simulink model "TV2016"  (Simulink 8.5)
settings: Solver=FixedStepDiscrete  StartTime=0.0  StopTime=inf  FixedStep=0.001  RelTol=1e-3
PreLoadFcn:
  | FSE_Parameters
values from neighbouring files (symbols this model uses):
  car_params = Simulink_Car_params    [TV2016_parameters.m]
  i_Diff = 15.47    [TV2016_parameters.m]
  Kp = 1    [TV2016_parameters.m]
  powerLimitControl = Simulink_el    [TV2016_parameters.m]
  settings = Simulink_Settings    [TV2016_parameters.m]
  SpdC_BCC = 0    [TV2016_parameters.m]
  Speed_Neg_sat = -21    [TV2016_parameters.m]
  Speed_Pos_sat = 21    [TV2016_parameters.m]
  speedEstimation = Simulink_speedEst    [TV2016_parameters.m]
  Tn_n = 0    [TV2016_parameters.m]
  tractionControl = Simulink_tc    [TV2016_parameters.m]
  Use_Joystick = 1    [TV2016_parameters.m]
  yawRateControl = Simulink_yawRate    [TV2016_parameters.m]
libraries: CarMaker4SL x174, simulink x27, simulink_extras x14
(part 4 of 5)

== system TV2016/CarMaker/IPG Vehicle/CarAndTrailer/Trailer/CreateBus Vhcl.Wheel.RR ==
  In1 : Inport
  Bus Creator3 : BusCreator  Inputs=14
  Demux3 : Demux  Outputs=14
  Out1 : Outport
  wires:
  Demux3/14 -> Bus Creator3/14  "Vhcl Wheel RR Trq_WhlBearing"
  Demux3/13 -> Bus Creator3/13  "Vhcl Wheel RR Trq_T2W"
  Demux3/12 -> Bus Creator3/12  "Vhcl Wheel RR SideSlip"
  Demux3/11 -> Bus Creator3/11  "Vhcl Wheel RR LongSlip"
  Demux3/10 -> Bus Creator3/10  "Vhcl Wheel RR vBelt"
  Demux3/9 -> Bus Creator3/9  "Vhcl Wheel RR Fz"
  Demux3/8 -> Bus Creator3/8  "Vhcl Wheel RR Fy"
  Demux3/7 -> Bus Creator3/7  "Vhcl Wheel RR Fx"
  Demux3/6 -> Bus Creator3/6  "Vhcl Wheel RR r_zxy z"
  Demux3/5 -> Bus Creator3/5  "Vhcl Wheel RR r_zxy y"
  Demux3/4 -> Bus Creator3/4  "Vhcl Wheel RR r_zxy x"
  Demux3/3 -> Bus Creator3/3  "Vhcl Wheel RR t z"
  Demux3/2 -> Bus Creator3/2  "Vhcl Wheel RR t y"
  In1/1 -> Demux3/1
  Bus Creator3/1 -> Out1/1
  Demux3/1 -> Bus Creator3/1  "Vhcl Wheel RR t x"

== system TV2016/CarMaker/IPG Vehicle/PowerTrain/Electric Powertrain/AMK FL ==
  Motor_speed_ref_in_RPM : Inport
  Whl_speed_rad_per_sec : Inport  Port=2
  "Torque_limit_pos " : Inport  Port=3
  Torque_limit_neg : Inport  Port=4
  Convert to RPM : Gain  Gain=60/(2*pi)
  Delay : Delay  DelayLength=3  InitialCondition=0
  Gain2 : Gain  Gain=-1
  Gear ratio : Gain  Gain=i_Diff
  Gear ratio2 : Gain  Gain=i_Diff
  Maximum torque output based on motor RPM : Lookup_n-D  NumberOfTableDimensions=1  BreakpointsForDimension1=[0,15000, 20000, 20500]  BreakpointsForDimension1Min=[0]  BreakpointsForDimension1Max=[20000]  Table=[21 21, 15, 0]  ExtrapMethod=Clip  UseLastTableValue=on  InternalRulePriority=Speed  OutMin=[0]  OutMax=[21]  RndMeth=Simplest  InputSameDT=on
  Saturation : simulink/Discontinuities/Saturation Dynamic  OutMin=[]  OutMax=[]  OutDataTypeStr=Inherit: Same as second input  OutDataType=fixdt(1, 16)  OutScaling=2^-10  DoSatur=off
  Saturation Dynamic1 : simulink/Discontinuities/Saturation Dynamic  OutMin=[]  OutMax=[]  OutDataTypeStr=Inherit: Same as second input  OutDataType=fixdt(1, 16)  OutScaling=2^-10  DoSatur=off
  Speed PI 1 : simulink/Continuous/PID Controller  Controller=PI  TimeDomain=Discrete-time  SampleTime=-1  IntegratorMethod=Forward Euler  FilterMethod=Forward Euler  Form=Parallel  UseFilter=on  ControllerParametersSource=internal  P=Kp  I=Tn_n  D=0  N=100  InitialConditionSource=internal  InitialConditionForIntegrator=0  InitialConditionForFilter=0  ExternalReset=none  LimitOutput=on  UpperSaturationLimit=Speed_Pos_sat  LowerSaturationLimit=Speed_Neg_sat  LinearizeAsGain=off  AntiWindupMode=back-calculation  Kb=SpdC_BCC  TrackingMode=off  Kt=1  PParamMin=[]  PParamMax=[]  IParamMin=[]  IParamMax=[]  DParamMin=[]  DParamMax=[]  NParamMin=[]  NParamMax=[]  KbParamMin=[]  KbParamMax=[]  KtParamMin=[]  KtParamMax=[]  POutMin=[]  POutMax=[]  IOutMin=[]  IOutMax=[]  DOutMin=[]  DOutMax=[]  NOutMin=[]  NOutMax=[]  KbOutMin=[]  KbOutMax=[]  KtOutMin=[]  KtOutMax=[]  IntegratorOutMin=[]  IntegratorOutMax=[]  FilterOutMin=[]  FilterOutMax=[]  SumOutMin=[]  SumOutMax=[]  SumI1OutMin=[]  SumI1OutMax=[]  SumI2OutMin=[]  SumI2OutMax=[]  SumI3OutMin=[]  SumI3OutMax=[]  SumDOutMin=[]  SumDOutMax=[]  SaturationOutMin=[]  SaturationOutMax=[]  IntegratorContinuousStateAttributes=''  IntegratorStateMustResolveToSignalObject=off  IntegratorRTWStateStorageClass=Auto  FilterContinuousStateAttributes=''  FilterStateMustResolveToSignalObject=off  FilterRTWStateStorageClass=Auto  DifferentiatorICPrevScaledInput=0  DifferentiatorOutMin=[]  DifferentiatorOutMax=[]
  Sum : Sum  Inputs=|+-
  "Torque_output_at_wheel " : Outport
  wires:
  Gear ratio/1 -> Convert to RPM/1
  Convert to RPM/1 -> Sum/2, Maximum torque output based on motor RPM/1
  Sum/1 -> Speed PI 1/1
  Saturation/1 -> Saturation Dynamic1/2
  Motor_speed_ref_in_RPM/1 -> Sum/1
  Torque_limit_neg/1 -> Saturation/3
  "Torque_limit_pos "/1 -> Saturation/1
  Gear ratio2/1 -> Delay/1
  Gain2/1 -> Saturation Dynamic1/3
  Whl_speed_rad_per_sec/1 -> Gear ratio/1
  Saturation Dynamic1/1 -> Gear ratio2/1
  Maximum torque output based on motor RPM/1 -> Gain2/1, Saturation Dynamic1/1
  Speed PI 1/1 -> Saturation/2
  Delay/1 -> "Torque_output_at_wheel "/1

== system TV2016/CarMaker/IPG Vehicle/PowerTrain/Electric Powertrain/AMK FR ==
  Motor_speed_ref_in_RPM : Inport
  Whl_speed_rad_per_sec : Inport  Port=2
  "Torque_limit_pos " : Inport  Port=3
  Torque_limit_neg : Inport  Port=4
  Convert to RPM : Gain  Gain=60/(2*pi)
  Delay : Delay  DelayLength=3  InitialCondition=0
  Gain2 : Gain  Gain=-1
  Gear ratio : Gain  Gain=i_Diff
  Gear ratio2 : Gain  Gain=i_Diff
  Maximum torque output based on motor RPM : Lookup_n-D  NumberOfTableDimensions=1  BreakpointsForDimension1=[0,15000, 20000, 20500]  BreakpointsForDimension1Min=[0]  BreakpointsForDimension1Max=[20000]  Table=[21 21, 15, 0]  ExtrapMethod=Clip  UseLastTableValue=on  InternalRulePriority=Speed  OutMin=[0]  OutMax=[21]  RndMeth=Simplest  InputSameDT=on
  Saturation : simulink/Discontinuities/Saturation Dynamic  OutMin=[]  OutMax=[]  OutDataTypeStr=Inherit: Same as second input  OutDataType=fixdt(1, 16)  OutScaling=2^-10  DoSatur=off
  Saturation Dynamic1 : simulink/Discontinuities/Saturation Dynamic  OutMin=[]  OutMax=[]  OutDataTypeStr=Inherit: Same as second input  OutDataType=fixdt(1, 16)  OutScaling=2^-10  DoSatur=off
  Speed PI 1 : simulink/Continuous/PID Controller  Controller=PI  TimeDomain=Discrete-time  SampleTime=-1  IntegratorMethod=Forward Euler  FilterMethod=Forward Euler  Form=Parallel  UseFilter=on  ControllerParametersSource=internal  P=Kp  I=Tn_n  D=0  N=100  InitialConditionSource=internal  InitialConditionForIntegrator=0  InitialConditionForFilter=0  ExternalReset=none  LimitOutput=on  UpperSaturationLimit=Speed_Pos_sat  LowerSaturationLimit=Speed_Neg_sat  LinearizeAsGain=off  AntiWindupMode=back-calculation  Kb=SpdC_BCC  TrackingMode=off  Kt=1  PParamMin=[]  PParamMax=[]  IParamMin=[]  IParamMax=[]  DParamMin=[]  DParamMax=[]  NParamMin=[]  NParamMax=[]  KbParamMin=[]  KbParamMax=[]  KtParamMin=[]  KtParamMax=[]  POutMin=[]  POutMax=[]  IOutMin=[]  IOutMax=[]  DOutMin=[]  DOutMax=[]  NOutMin=[]  NOutMax=[]  KbOutMin=[]  KbOutMax=[]  KtOutMin=[]  KtOutMax=[]  IntegratorOutMin=[]  IntegratorOutMax=[]  FilterOutMin=[]  FilterOutMax=[]  SumOutMin=[]  SumOutMax=[]  SumI1OutMin=[]  SumI1OutMax=[]  SumI2OutMin=[]  SumI2OutMax=[]  SumI3OutMin=[]  SumI3OutMax=[]  SumDOutMin=[]  SumDOutMax=[]  SaturationOutMin=[]  SaturationOutMax=[]  IntegratorContinuousStateAttributes=''  IntegratorStateMustResolveToSignalObject=off  IntegratorRTWStateStorageClass=Auto  FilterContinuousStateAttributes=''  FilterStateMustResolveToSignalObject=off  FilterRTWStateStorageClass=Auto  DifferentiatorICPrevScaledInput=0  DifferentiatorOutMin=[]  DifferentiatorOutMax=[]
  Sum : Sum  Inputs=|+-
  "Torque_Output " : Outport
  wires:
  Gear ratio/1 -> Convert to RPM/1
  Convert to RPM/1 -> Maximum torque output based on motor RPM/1, Sum/2
  Sum/1 -> Speed PI 1/1
  Saturation/1 -> Saturation Dynamic1/2
  Motor_speed_ref_in_RPM/1 -> Sum/1
  Torque_limit_neg/1 -> Saturation/3
  "Torque_limit_pos "/1 -> Saturation/1
  Gear ratio2/1 -> Delay/1
  Gain2/1 -> Saturation Dynamic1/3
  Whl_speed_rad_per_sec/1 -> Gear ratio/1
  Saturation Dynamic1/1 -> Gear ratio2/1
  Maximum torque output based on motor RPM/1 -> Gain2/1, Saturation Dynamic1/1
  Speed PI 1/1 -> Saturation/2
  Delay/1 -> "Torque_Output "/1

== system TV2016/CarMaker/IPG Vehicle/PowerTrain/Electric Powertrain/AMK RL ==
  Motor_speed_ref_in_RPM : Inport
  Whl_speed_rad_per_sec : Inport  Port=2
  "Torque_limit_pos " : Inport  Port=3
  Torque_limit_neg : Inport  Port=4
  Convert to RPM : Gain  Gain=60/(2*pi)
  Delay : Delay  DelayLength=3  InitialCondition=0
  Gain2 : Gain  Gain=-1
  Gear ratio : Gain  Gain=i_Diff
  Gear ratio2 : Gain  Gain=i_Diff
  Maximum torque output based on motor RPM : Lookup_n-D  NumberOfTableDimensions=1  BreakpointsForDimension1=[0,15000, 20000, 20500]  BreakpointsForDimension1Min=[0]  BreakpointsForDimension1Max=[20000]  Table=[21 21, 15, 0]  ExtrapMethod=Clip  UseLastTableValue=on  InternalRulePriority=Speed  OutMin=[0]  OutMax=[21]  RndMeth=Simplest  InputSameDT=on
  Saturation : simulink/Discontinuities/Saturation Dynamic  OutMin=[]  OutMax=[]  OutDataTypeStr=Inherit: Same as second input  OutDataType=fixdt(1, 16)  OutScaling=2^-10  DoSatur=off
  Saturation Dynamic1 : simulink/Discontinuities/Saturation Dynamic  OutMin=[]  OutMax=[]  OutDataTypeStr=Inherit: Same as second input  OutDataType=fixdt(1, 16)  OutScaling=2^-10  DoSatur=off
  Speed PI 1 : simulink/Continuous/PID Controller  Controller=PI  TimeDomain=Discrete-time  SampleTime=-1  IntegratorMethod=Forward Euler  FilterMethod=Forward Euler  Form=Parallel  UseFilter=on  ControllerParametersSource=internal  P=Kp  I=Tn_n  D=0  N=100  InitialConditionSource=internal  InitialConditionForIntegrator=0  InitialConditionForFilter=0  ExternalReset=none  LimitOutput=on  UpperSaturationLimit=Speed_Pos_sat  LowerSaturationLimit=Speed_Neg_sat  LinearizeAsGain=off  AntiWindupMode=back-calculation  Kb=SpdC_BCC  TrackingMode=off  Kt=1  PParamMin=[]  PParamMax=[]  IParamMin=[]  IParamMax=[]  DParamMin=[]  DParamMax=[]  NParamMin=[]  NParamMax=[]  KbParamMin=[]  KbParamMax=[]  KtParamMin=[]  KtParamMax=[]  POutMin=[]  POutMax=[]  IOutMin=[]  IOutMax=[]  DOutMin=[]  DOutMax=[]  NOutMin=[]  NOutMax=[]  KbOutMin=[]  KbOutMax=[]  KtOutMin=[]  KtOutMax=[]  IntegratorOutMin=[]  IntegratorOutMax=[]  FilterOutMin=[]  FilterOutMax=[]  SumOutMin=[]  SumOutMax=[]  SumI1OutMin=[]  SumI1OutMax=[]  SumI2OutMin=[]  SumI2OutMax=[]  SumI3OutMin=[]  SumI3OutMax=[]  SumDOutMin=[]  SumDOutMax=[]  SaturationOutMin=[]  SaturationOutMax=[]  IntegratorContinuousStateAttributes=''  IntegratorStateMustResolveToSignalObject=off  IntegratorRTWStateStorageClass=Auto  FilterContinuousStateAttributes=''  FilterStateMustResolveToSignalObject=off  FilterRTWStateStorageClass=Auto  DifferentiatorICPrevScaledInput=0  DifferentiatorOutMin=[]  DifferentiatorOutMax=[]
  Sum : Sum  Inputs=|+-
  "Torque_Output " : Outport
  wires:
  Delay/1 -> "Torque_Output "/1
  Speed PI 1/1 -> Saturation/2
  Maximum torque output based on motor RPM/1 -> Saturation Dynamic1/1, Gain2/1
  Saturation Dynamic1/1 -> Gear ratio2/1
  Whl_speed_rad_per_sec/1 -> Gear ratio/1
  Gain2/1 -> Saturation Dynamic1/3
  Gear ratio2/1 -> Delay/1
  "Torque_limit_pos "/1 -> Saturation/1
  Torque_limit_neg/1 -> Saturation/3
  Motor_speed_ref_in_RPM/1 -> Sum/1
  Saturation/1 -> Saturation Dynamic1/2
  Sum/1 -> Speed PI 1/1
  Convert to RPM/1 -> Sum/2, Maximum torque output based on motor RPM/1
  Gear ratio/1 -> Convert to RPM/1

== system TV2016/CarMaker/IPG Vehicle/PowerTrain/Electric Powertrain/AMK RR ==
  Motor_speed_ref_in_RPM : Inport
  Whl_speed_rad_per_sec : Inport  Port=2
  "Torque_limit_pos " : Inport  Port=3
  Torque_limit_neg : Inport  Port=4
  Convert to RPM : Gain  Gain=60/(2*pi)
  Delay : Delay  DelayLength=3  InitialCondition=0
  Gain2 : Gain  Gain=-1
  Gear ratio : Gain  Gain=i_Diff
  Gear ratio2 : Gain  Gain=i_Diff
  Maximum torque output based on motor RPM : Lookup_n-D  NumberOfTableDimensions=1  BreakpointsForDimension1=[0,15000, 20000, 20500]  BreakpointsForDimension1Min=[0]  BreakpointsForDimension1Max=[20000]  Table=[21 21, 15, 0]  ExtrapMethod=Clip  UseLastTableValue=on  InternalRulePriority=Speed  OutMin=[0]  OutMax=[21]  RndMeth=Simplest  InputSameDT=on
  Saturation : simulink/Discontinuities/Saturation Dynamic  OutMin=[]  OutMax=[]  OutDataTypeStr=Inherit: Same as second input  OutDataType=fixdt(1, 16)  OutScaling=2^-10  DoSatur=off
  Saturation Dynamic1 : simulink/Discontinuities/Saturation Dynamic  OutMin=[]  OutMax=[]  OutDataTypeStr=Inherit: Same as second input  OutDataType=fixdt(1, 16)  OutScaling=2^-10  DoSatur=off
  Speed PI 1 : simulink/Continuous/PID Controller  Controller=PI  TimeDomain=Discrete-time  SampleTime=-1  IntegratorMethod=Forward Euler  FilterMethod=Forward Euler  Form=Parallel  UseFilter=on  ControllerParametersSource=internal  P=Kp  I=Tn_n  D=0  N=100  InitialConditionSource=internal  InitialConditionForIntegrator=0  InitialConditionForFilter=0  ExternalReset=none  LimitOutput=on  UpperSaturationLimit=Speed_Pos_sat  LowerSaturationLimit=Speed_Neg_sat  LinearizeAsGain=off  AntiWindupMode=back-calculation  Kb=SpdC_BCC  TrackingMode=off  Kt=1  PParamMin=[]  PParamMax=[]  IParamMin=[]  IParamMax=[]  DParamMin=[]  DParamMax=[]  NParamMin=[]  NParamMax=[]  KbParamMin=[]  KbParamMax=[]  KtParamMin=[]  KtParamMax=[]  POutMin=[]  POutMax=[]  IOutMin=[]  IOutMax=[]  DOutMin=[]  DOutMax=[]  NOutMin=[]  NOutMax=[]  KbOutMin=[]  KbOutMax=[]  KtOutMin=[]  KtOutMax=[]  IntegratorOutMin=[]  IntegratorOutMax=[]  FilterOutMin=[]  FilterOutMax=[]  SumOutMin=[]  SumOutMax=[]  SumI1OutMin=[]  SumI1OutMax=[]  SumI2OutMin=[]  SumI2OutMax=[]  SumI3OutMin=[]  SumI3OutMax=[]  SumDOutMin=[]  SumDOutMax=[]  SaturationOutMin=[]  SaturationOutMax=[]  IntegratorContinuousStateAttributes=''  IntegratorStateMustResolveToSignalObject=off  IntegratorRTWStateStorageClass=Auto  FilterContinuousStateAttributes=''  FilterStateMustResolveToSignalObject=off  FilterRTWStateStorageClass=Auto  DifferentiatorICPrevScaledInput=0  DifferentiatorOutMin=[]  DifferentiatorOutMax=[]
  Sum : Sum  Inputs=|+-
  "Torque_Output " : Outport
  wires:
  Gear ratio/1 -> Convert to RPM/1
  Convert to RPM/1 -> Maximum torque output based on motor RPM/1, Sum/2
  Sum/1 -> Speed PI 1/1
  Saturation/1 -> Saturation Dynamic1/2
  Motor_speed_ref_in_RPM/1 -> Sum/1
  Torque_limit_neg/1 -> Saturation/3
  "Torque_limit_pos "/1 -> Saturation/1
  Gear ratio2/1 -> Delay/1
  Gain2/1 -> Saturation Dynamic1/3
  Whl_speed_rad_per_sec/1 -> Gear ratio/1
  Saturation Dynamic1/1 -> Gear ratio2/1
  Maximum torque output based on motor RPM/1 -> Gain2/1, Saturation Dynamic1/1
  Speed PI 1/1 -> Saturation/2
  Delay/1 -> "Torque_Output "/1

== system TV2016/CarMaker/Control_System /Control /Slip Rate Control /SMC Traction Control/Slip Rate FL ==
  SR_ref : Inport
  Kp : Inport  Port=2
  SR : Inport  Port=3
  states : Inport  Port=4
  SMC : MATLAB Function  TreatAsAtomicUnit=on
  mu lookup : Lookup_n-D  NumberOfTableDimensions=1  BreakpointsForDimension1="[0  0.15 1]"  Table=[0 1.5 0.75]  ExtrapMethod=Clip  UseLastTableValue=on  InternalRulePriority=Speed  RndMeth=Simplest  InputSameDT=on
  Tc : Outport
  wires:
  SR_ref/1 -> SMC/3(SR_ref)
  SR/1 -> SMC/2(SR), mu lookup/1
  mu lookup/1 -> SMC/1(muOfSlip)
  Kp/1 -> SMC/5(K)
  states/1 -> SMC/4(states)
  SMC/1(TC) -> Tc/1

== system TV2016/CarMaker/Control_System /Control /Slip Rate Control /SMC Traction Control/Slip Rate FL1 ==
  SR_ref : Inport
  Kp : Inport  Port=2
  SR : Inport  Port=3
  states : Inport  Port=4
  SMC : MATLAB Function  TreatAsAtomicUnit=on
  mu lookup : Lookup_n-D  NumberOfTableDimensions=1  BreakpointsForDimension1="[0  0.15 1]"  Table=[0 1.5 0.75]  ExtrapMethod=Clip  UseLastTableValue=on  InternalRulePriority=Speed  RndMeth=Simplest  InputSameDT=on
  Tc : Outport
  wires:
  SMC/1(TC) -> Tc/1
  states/1 -> SMC/4(states)
  Kp/1 -> SMC/5(K)
  mu lookup/1 -> SMC/1(muOfSlip)
  SR/1 -> mu lookup/1, SMC/2(SR)
  SR_ref/1 -> SMC/3(SR_ref)

== system TV2016/CarMaker/Control_System /Control /Slip Rate Control /SMC Traction Control/Slip Rate FL2 ==
  SR_ref : Inport
  Kp : Inport  Port=2
  SR : Inport  Port=3
  states : Inport  Port=4
  SMC : MATLAB Function  TreatAsAtomicUnit=on
  mu lookup : Lookup_n-D  NumberOfTableDimensions=1  BreakpointsForDimension1="[0  0.15 1]"  Table=[0 1.5 0.75]  ExtrapMethod=Clip  UseLastTableValue=on  InternalRulePriority=Speed  RndMeth=Simplest  InputSameDT=on
  Tc : Outport
  wires:
  SR_ref/1 -> SMC/3(SR_ref)
  SR/1 -> SMC/2(SR), mu lookup/1
  mu lookup/1 -> SMC/1(muOfSlip)
  Kp/1 -> SMC/5(K)
  states/1 -> SMC/4(states)
  SMC/1(TC) -> Tc/1

== system TV2016/CarMaker/Control_System /Control /Slip Rate Control /SMC Traction Control/Slip Rate FL3 ==
  SR_ref : Inport
  Kp : Inport  Port=2
  SR : Inport  Port=3
  states : Inport  Port=4
  SMC : MATLAB Function  TreatAsAtomicUnit=on
  mu lookup : Lookup_n-D  NumberOfTableDimensions=1  BreakpointsForDimension1="[0  0.15 1]"  Table=[0 1.5 0.75]  ExtrapMethod=Clip  UseLastTableValue=on  InternalRulePriority=Speed  RndMeth=Simplest  InputSameDT=on
  Tc : Outport
  wires:
  SMC/1(TC) -> Tc/1
  states/1 -> SMC/4(states)
  Kp/1 -> SMC/5(K)
  mu lookup/1 -> SMC/1(muOfSlip)
  SR/1 -> mu lookup/1, SMC/2(SR)
  SR_ref/1 -> SMC/3(SR_ref)

== system TV2016/CarMaker/Control_System /Control /Slip Rate Control /Traction Controllers/Slip Rate FL ==
  SR_ref : Inport
  Kp : Inport  Port=2
  Ki : Inport  Port=3
  SR : Inport  Port=4
  Ti_ref : Inport  Port=5
  Constant : Constant  Value=single(0)
  Constant1 : Constant  Value=single(0)
  Discrete-Time Integrator2 : DiscreteIntegrator  ExternalReset=either  InitialConditionSetting=State (most efficient)  SampleTime=-1
  Gain : Gain  Gain=single(-1)
  Gain1 : Gain  Gain=single(-1)
  Gain2 : Gain  Gain=tractionControl.Kb
  Gain7 : Gain  Gain=single(-1)
  Product : Product
  Product1 : Product
  Saturation Dynamic : simulink/Discontinuities/Saturation Dynamic  OutMin=[]  OutMax=[]  OutDataTypeStr=single  OutputDataTypeScalingMode=single  OutDataType=fixdt(1, 16)  OutScaling=2^-10  DoSatur=off
  Saturation Dynamic1 : simulink/Discontinuities/Saturation Dynamic  OutMin=[]  OutMax=[]  OutDataTypeStr=single  OutputDataTypeScalingMode=single  OutDataType=fixdt(1, 16)  OutScaling=2^-10  DoSatur=off
  Sum : Sum  Inputs=|+-
  Sum1 : Sum  Inputs=++|
  Sum2 : Sum  Inputs=|++
  Sum3 : Sum  Inputs=|+-  AccumDataTypeStr=single
  Switch : Switch  Criteria=u2 > Threshold
  Switch1 : Switch  Criteria=u2 > Threshold
  Switch2 : Switch  Criteria=u2 > Threshold
  TC_output : Outport
  wires:
  SR/1 -> Sum/2
  Product/1 -> Sum2/2
  Saturation Dynamic/1 -> Sum2/1, Sum3/1
  Sum/1 -> Product/2, Product1/2
  Gain1/1 -> Switch1/1
  Constant1/1 -> Switch1/3
  Constant/1 -> Switch/1
  Gain/1 -> Switch/3
  Ti_ref/1 -> Discrete-Time Integrator2/2, Switch2/2, Switch1/2, Gain1/1, Gain/1, Switch/2
  SR_ref/1 -> Gain7/1, Switch2/1
  Gain7/1 -> Switch2/3
  Switch2/1 -> Sum/1
  Switch/1 -> Saturation Dynamic1/1, Saturation Dynamic/1
  Switch1/1 -> Saturation Dynamic1/3, Saturation Dynamic/3
  Kp/1 -> Product/1
  Sum1/1 -> Discrete-Time Integrator2/1
  Ki/1 -> Product1/1
  Product1/1 -> Sum1/2
  Discrete-Time Integrator2/1 -> Saturation Dynamic/2, Sum3/2
  Sum3/1 -> Gain2/1
  Gain2/1 -> Sum1/1
  Sum2/1 -> Saturation Dynamic1/2
  Saturation Dynamic1/1 -> TC_output/1

== system TV2016/CarMaker/Control_System /Control /Slip Rate Control /Traction Controllers/Slip Rate FR ==
  SR_ref : Inport
  Kp : Inport  Port=2
  Ki : Inport  Port=3
  SR : Inport  Port=4
  Ti_ref : Inport  Port=5
  Constant : Constant  Value=single(0)
  Constant1 : Constant  Value=single(0)
  Discrete-Time Integrator2 : DiscreteIntegrator  ExternalReset=either  InitialConditionSetting=State (most efficient)  SampleTime=-1
  Gain : Gain  Gain=single(-1)
  Gain1 : Gain  Gain=single(-1)
  Gain2 : Gain  Gain=tractionControl.Kb
  Gain7 : Gain  Gain=single(-1)
  PI_Kp 1 : Scope
      settings: ShowLegends=on  YMin=333.5  YMax=341  SaveName=ScopeData39
  PI_Kp 2 : Scope
      settings: ShowLegends=on  YMin=333.5  YMax=341  SaveName=ScopeData40
  PI_Kp 4 : Scope
      settings: ShowLegends=on  YMin=333.5  YMax=341  SaveName=ScopeData34
  Product : Product
  Product1 : Product
  Saturation Dynamic : simulink/Discontinuities/Saturation Dynamic  OutMin=[]  OutMax=[]  OutDataTypeStr=single  OutputDataTypeScalingMode=single  OutDataType=fixdt(1, 16)  OutScaling=2^-10  DoSatur=off
  Saturation Dynamic1 : simulink/Discontinuities/Saturation Dynamic  OutMin=[]  OutMax=[]  OutDataTypeStr=single  OutputDataTypeScalingMode=single  OutDataType=fixdt(1, 16)  OutScaling=2^-10  DoSatur=off
  Sum : Sum  Inputs=|+-
  Sum1 : Sum  Inputs=++|
  Sum2 : Sum  Inputs=|++
  Sum3 : Sum  Inputs=|+-  AccumDataTypeStr=single
  Switch : Switch  Criteria=u2 > Threshold
  Switch1 : Switch  Criteria=u2 > Threshold
  Switch2 : Switch  Criteria=u2 > Threshold
  integrator : Scope
      settings: ShowLegends=on  YMin=333.5  YMax=341  SaveName=ScopeData42
  TC_output : Outport
  wires:
  Saturation Dynamic1/1 -> TC_output/1, PI_Kp 1/1
  Sum2/1 -> Saturation Dynamic1/2
  Gain2/1 -> PI_Kp 4/1, Sum1/1
  Sum3/1 -> Gain2/1
  Discrete-Time Integrator2/1 -> Sum3/2, Saturation Dynamic/2, integrator/1
  Product1/1 -> Sum1/2
  Ki/1 -> Product1/1
  Sum1/1 -> Discrete-Time Integrator2/1
  Kp/1 -> Product/1
  Switch1/1 -> Saturation Dynamic/3, Saturation Dynamic1/3
  Switch/1 -> Saturation Dynamic/1, Saturation Dynamic1/1
  Switch2/1 -> Sum/1
  Gain7/1 -> Switch2/3
  SR_ref/1 -> Switch2/1, Gain7/1
  Ti_ref/1 -> Switch2/2, Discrete-Time Integrator2/2, Switch/2, Gain/1, Gain1/1, Switch1/2
  Gain/1 -> Switch/3
  Constant/1 -> Switch/1
  Constant1/1 -> Switch1/3
  Gain1/1 -> Switch1/1
  Sum/1 -> Product1/2, Product/2
  Saturation Dynamic/1 -> Sum3/1, Sum2/1
  Product/1 -> Sum2/2, PI_Kp 2/1
  SR/1 -> Sum/2

== system TV2016/CarMaker/Control_System /Control /Slip Rate Control /Traction Controllers/Slip Rate RL ==
  SR_ref : Inport
  Kp : Inport  Port=2
  Ki : Inport  Port=3
  SR : Inport  Port=4
  Ti_ref : Inport  Port=5
  Constant : Constant  Value=single(0)
  Constant1 : Constant  Value=single(0)
  Discrete-Time Integrator2 : DiscreteIntegrator  ExternalReset=either  InitialConditionSetting=State (most efficient)  SampleTime=-1
  Gain : Gain  Gain=single(-1)
  Gain1 : Gain  Gain=single(-1)
  Gain2 : Gain  Gain=tractionControl.Kb
  Gain7 : Gain  Gain=single(-1)
  PI_Kp 1 : Scope
      settings: ShowLegends=on  YMin=333.5  YMax=341  SaveName=ScopeData39
  PI_Kp 2 : Scope
      settings: ShowLegends=on  YMin=333.5  YMax=341  SaveName=ScopeData40
  PI_Kp 4 : Scope
      settings: ShowLegends=on  YMin=333.5  YMax=341  SaveName=ScopeData34
  Product : Product
  Product1 : Product
  Saturation Dynamic : simulink/Discontinuities/Saturation Dynamic  OutMin=[]  OutMax=[]  OutDataTypeStr=single  OutputDataTypeScalingMode=single  OutDataType=fixdt(1, 16)  OutScaling=2^-10  DoSatur=off
  Saturation Dynamic1 : simulink/Discontinuities/Saturation Dynamic  OutMin=[]  OutMax=[]  OutDataTypeStr=single  OutputDataTypeScalingMode=single  OutDataType=fixdt(1, 16)  OutScaling=2^-10  DoSatur=off
  Sum : Sum  Inputs=|+-
  Sum1 : Sum  Inputs=++|
  Sum2 : Sum  Inputs=|++
  Sum3 : Sum  Inputs=|+-  AccumDataTypeStr=single
  Switch : Switch  Criteria=u2 > Threshold
  Switch1 : Switch  Criteria=u2 > Threshold
  Switch2 : Switch  Criteria=u2 > Threshold
  integrator : Scope
      settings: ShowLegends=on  YMin=333.5  YMax=341  SaveName=ScopeData42
  TC_output : Outport
  wires:
  Saturation Dynamic1/1 -> TC_output/1, PI_Kp 1/1
  Sum2/1 -> Saturation Dynamic1/2
  Gain2/1 -> PI_Kp 4/1, Sum1/1
  Sum3/1 -> Gain2/1
  Discrete-Time Integrator2/1 -> Sum3/2, Saturation Dynamic/2, integrator/1
  Product1/1 -> Sum1/2
  Ki/1 -> Product1/1
  Sum1/1 -> Discrete-Time Integrator2/1
  Kp/1 -> Product/1
  Switch1/1 -> Saturation Dynamic/3, Saturation Dynamic1/3
  Switch/1 -> Saturation Dynamic/1, Saturation Dynamic1/1
  Switch2/1 -> Sum/1
  Gain7/1 -> Switch2/3
  SR_ref/1 -> Switch2/1, Gain7/1
  Ti_ref/1 -> Switch2/2, Discrete-Time Integrator2/2, Switch/2, Gain/1, Gain1/1, Switch1/2
  Gain/1 -> Switch/3
  Constant/1 -> Switch/1
  Constant1/1 -> Switch1/3
  Gain1/1 -> Switch1/1
  Sum/1 -> Product1/2, Product/2
  Saturation Dynamic/1 -> Sum3/1, Sum2/1
  Product/1 -> Sum2/2, PI_Kp 2/1
  SR/1 -> Sum/2

== system TV2016/CarMaker/Control_System /Control /Slip Rate Control /Traction Controllers/Slip Rate RR ==
  SR_ref : Inport
  Kp : Inport  Port=2
  Ki : Inport  Port=3
  SR : Inport  Port=4
  Ti_ref : Inport  Port=5
  Constant : Constant  Value=single(0)
  Constant1 : Constant  Value=single(0)
  Discrete-Time Integrator2 : DiscreteIntegrator  ExternalReset=either  InitialConditionSetting=State (most efficient)  SampleTime=-1
  Gain : Gain  Gain=single(-1)
  Gain1 : Gain  Gain=single(-1)
  Gain2 : Gain  Gain=tractionControl.Kb
  Gain7 : Gain  Gain=single(-1)
  PI_Kp 1 : Scope
      settings: ShowLegends=on  YMin=333.5  YMax=341  SaveName=ScopeData39
  PI_Kp 2 : Scope
      settings: ShowLegends=on  YMin=333.5  YMax=341  SaveName=ScopeData40
  PI_Kp 4 : Scope
      settings: ShowLegends=on  YMin=333.5  YMax=341  SaveName=ScopeData34
  Product : Product
  Product1 : Product
  Saturation Dynamic : simulink/Discontinuities/Saturation Dynamic  OutMin=[]  OutMax=[]  OutDataTypeStr=single  OutputDataTypeScalingMode=single  OutDataType=fixdt(1, 16)  OutScaling=2^-10  DoSatur=off
  Saturation Dynamic1 : simulink/Discontinuities/Saturation Dynamic  OutMin=[]  OutMax=[]  OutDataTypeStr=single  OutputDataTypeScalingMode=single  OutDataType=fixdt(1, 16)  OutScaling=2^-10  DoSatur=off
  Sum : Sum  Inputs=|+-
  Sum1 : Sum  Inputs=++|
  Sum2 : Sum  Inputs=|++
  Sum3 : Sum  Inputs=|+-  AccumDataTypeStr=single
  Switch : Switch  Criteria=u2 > Threshold
  Switch1 : Switch  Criteria=u2 > Threshold
  Switch2 : Switch  Criteria=u2 > Threshold
  integrator : Scope
      settings: ShowLegends=on  YMin=333.5  YMax=341  SaveName=ScopeData42
  TC_output : Outport
  wires:
  SR/1 -> Sum/2
  Product/1 -> PI_Kp 2/1, Sum2/2
  Saturation Dynamic/1 -> Sum2/1, Sum3/1
  Sum/1 -> Product/2, Product1/2
  Gain1/1 -> Switch1/1
  Constant1/1 -> Switch1/3
  Constant/1 -> Switch/1
  Gain/1 -> Switch/3
  Ti_ref/1 -> Switch1/2, Gain1/1, Gain/1, Switch/2, Discrete-Time Integrator2/2, Switch2/2
  SR_ref/1 -> Gain7/1, Switch2/1
  Gain7/1 -> Switch2/3
  Switch2/1 -> Sum/1
  Switch/1 -> Saturation Dynamic1/1, Saturation Dynamic/1
  Switch1/1 -> Saturation Dynamic1/3, Saturation Dynamic/3
  Kp/1 -> Product/1
  Sum1/1 -> Discrete-Time Integrator2/1
  Ki/1 -> Product1/1
  Product1/1 -> Sum1/2
  Discrete-Time Integrator2/1 -> integrator/1, Saturation Dynamic/2, Sum3/2
  Sum3/1 -> Gain2/1
  Gain2/1 -> Sum1/1, PI_Kp 4/1
  Sum2/1 -> Saturation Dynamic1/2
  Saturation Dynamic1/1 -> PI_Kp 1/1, TC_output/1

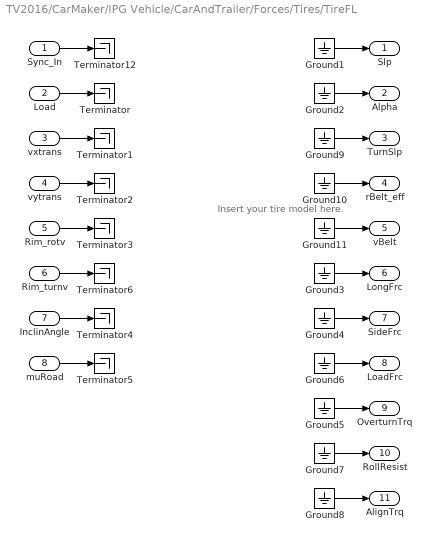
== system TV2016/CarMaker/IPG Vehicle/CarAndTrailer/Forces/Tires/TireFL ==
  note: Insert your tire model here.
  Sync_In : Inport
  Load : Inport  Port=2
  vxtrans : Inport  Port=3
  vytrans : Inport  Port=4
  Rim_rotv : Inport  Port=5
  Rim_turnv : Inport  Port=6
  InclinAngle : Inport  Port=7
  muRoad : Inport  Port=8
  Ground{1..11} (11 alike) : Ground
  Terminator{,1..6,12} (8 alike) : Terminator
  Slp : Outport
  Alpha : Outport  Port=2
  TurnSlp : Outport  Port=3
  rBelt_eff : Outport  Port=4
  vBelt : Outport  Port=5
  LongFrc : Outport  Port=6
  SideFrc : Outport  Port=7
  LoadFrc : Outport  Port=8
  OverturnTrq : Outport  Port=9
  RollResist : Outport  Port=10
  AlignTrq : Outport  Port=11
  wires:
  Ground11/1 -> vBelt/1
  Ground10/1 -> rBelt_eff/1
  Ground9/1 -> TurnSlp/1
  Rim_turnv/1 -> Terminator6/1
  Sync_In/1 -> Terminator12/1
  Ground2/1 -> Alpha/1
  Ground3/1 -> LongFrc/1
  Ground4/1 -> SideFrc/1
  Ground5/1 -> OverturnTrq/1
  vxtrans/1 -> Terminator1/1
  vytrans/1 -> Terminator2/1
  Rim_rotv/1 -> Terminator3/1
  InclinAngle/1 -> Terminator4/1
  muRoad/1 -> Terminator5/1
  Load/1 -> Terminator/1
  Ground1/1 -> Slp/1
  Ground6/1 -> LoadFrc/1
  Ground7/1 -> RollResist/1
  Ground8/1 -> AlignTrq/1

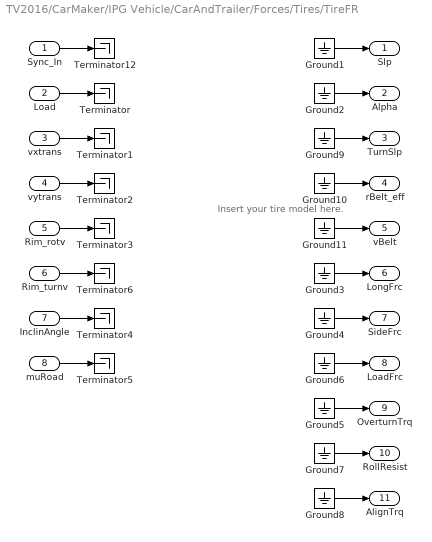
== system TV2016/CarMaker/IPG Vehicle/CarAndTrailer/Forces/Tires/TireFR ==
  note: Insert your tire model here.
  Sync_In : Inport
  Load : Inport  Port=2
  vxtrans : Inport  Port=3
  vytrans : Inport  Port=4
  Rim_rotv : Inport  Port=5
  Rim_turnv : Inport  Port=6
  InclinAngle : Inport  Port=7
  muRoad : Inport  Port=8
  Ground{1..11} (11 alike) : Ground
  Terminator{,1..6,12} (8 alike) : Terminator
  Slp : Outport
  Alpha : Outport  Port=2
  TurnSlp : Outport  Port=3
  rBelt_eff : Outport  Port=4
  vBelt : Outport  Port=5
  LongFrc : Outport  Port=6
  SideFrc : Outport  Port=7
  LoadFrc : Outport  Port=8
  OverturnTrq : Outport  Port=9
  RollResist : Outport  Port=10
  AlignTrq : Outport  Port=11
  wires:
  Ground11/1 -> vBelt/1
  Ground10/1 -> rBelt_eff/1
  Ground9/1 -> TurnSlp/1
  Rim_turnv/1 -> Terminator6/1
  Sync_In/1 -> Terminator12/1
  Ground2/1 -> Alpha/1
  Ground3/1 -> LongFrc/1
  Ground4/1 -> SideFrc/1
  Ground5/1 -> OverturnTrq/1
  vxtrans/1 -> Terminator1/1
  vytrans/1 -> Terminator2/1
  Rim_rotv/1 -> Terminator3/1
  InclinAngle/1 -> Terminator4/1
  muRoad/1 -> Terminator5/1
  Load/1 -> Terminator/1
  Ground1/1 -> Slp/1
  Ground6/1 -> LoadFrc/1
  Ground7/1 -> RollResist/1
  Ground8/1 -> AlignTrq/1

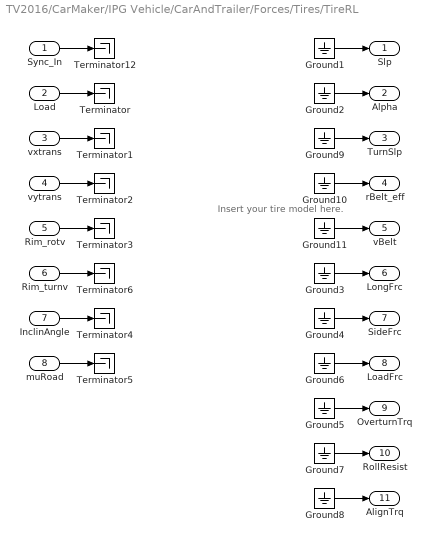
== system TV2016/CarMaker/IPG Vehicle/CarAndTrailer/Forces/Tires/TireRL ==
  note: Insert your tire model here.
  Sync_In : Inport
  Load : Inport  Port=2
  vxtrans : Inport  Port=3
  vytrans : Inport  Port=4
  Rim_rotv : Inport  Port=5
  Rim_turnv : Inport  Port=6
  InclinAngle : Inport  Port=7
  muRoad : Inport  Port=8
  Ground{1..11} (11 alike) : Ground
  Terminator{,1..6,12} (8 alike) : Terminator
  Slp : Outport
  Alpha : Outport  Port=2
  TurnSlp : Outport  Port=3
  rBelt_eff : Outport  Port=4
  vBelt : Outport  Port=5
  LongFrc : Outport  Port=6
  SideFrc : Outport  Port=7
  LoadFrc : Outport  Port=8
  OverturnTrq : Outport  Port=9
  RollResist : Outport  Port=10
  AlignTrq : Outport  Port=11
  wires:
  Ground11/1 -> vBelt/1
  Ground10/1 -> rBelt_eff/1
  Ground9/1 -> TurnSlp/1
  Rim_turnv/1 -> Terminator6/1
  Sync_In/1 -> Terminator12/1
  Ground2/1 -> Alpha/1
  Ground3/1 -> LongFrc/1
  Ground4/1 -> SideFrc/1
  Ground5/1 -> OverturnTrq/1
  vxtrans/1 -> Terminator1/1
  vytrans/1 -> Terminator2/1
  Rim_rotv/1 -> Terminator3/1
  InclinAngle/1 -> Terminator4/1
  muRoad/1 -> Terminator5/1
  Load/1 -> Terminator/1
  Ground1/1 -> Slp/1
  Ground6/1 -> LoadFrc/1
  Ground7/1 -> RollResist/1
  Ground8/1 -> AlignTrq/1

== system TV2016/CarMaker/IPG Vehicle/CarAndTrailer/Forces/Tires/TireRR ==
  note: Insert your tire model here.
  Sync_In : Inport
  Load : Inport  Port=2
  vxtrans : Inport  Port=3
  vytrans : Inport  Port=4
  Rim_rotv : Inport  Port=5
  Rim_turnv : Inport  Port=6
  InclinAngle : Inport  Port=7
  muRoad : Inport  Port=8
  Ground{1..11} (11 alike) : Ground
  Terminator{,1..6,12} (8 alike) : Terminator
  Slp : Outport
  Alpha : Outport  Port=2
  TurnSlp : Outport  Port=3
  rBelt_eff : Outport  Port=4
  vBelt : Outport  Port=5
  LongFrc : Outport  Port=6
  SideFrc : Outport  Port=7
  LoadFrc : Outport  Port=8
  OverturnTrq : Outport  Port=9
  RollResist : Outport  Port=10
  AlignTrq : Outport  Port=11
  wires:
  Ground11/1 -> vBelt/1
  Ground10/1 -> rBelt_eff/1
  Ground9/1 -> TurnSlp/1
  Rim_turnv/1 -> Terminator6/1
  Sync_In/1 -> Terminator12/1
  Ground2/1 -> Alpha/1
  Ground3/1 -> LongFrc/1
  Ground4/1 -> SideFrc/1
  Ground5/1 -> OverturnTrq/1
  vxtrans/1 -> Terminator1/1
  vytrans/1 -> Terminator2/1
  Rim_rotv/1 -> Terminator3/1
  InclinAngle/1 -> Terminator4/1
  muRoad/1 -> Terminator5/1
  Load/1 -> Terminator/1
  Ground1/1 -> Slp/1
  Ground6/1 -> LoadFrc/1
  Ground7/1 -> RollResist/1
  Ground8/1 -> AlignTrq/1

== matlab function CarMaker/Control_System /Control /Power Limit Torque Reduction Controller /extractPower ==
  data: states input double; power output double; powerLimitControl parameter double
function power = extractPower(states,powerLimitControl)
%#codegen


if (powerLimitControl.enable == uint32(1))
    power = states.power;
else
    power = single(0);
end

end

== matlab function CarMaker/Control_System /Control /Yaw Rate Controller /yawRateReference ==
  data: r_der_error output double; r_error output double; vx output double; states input Bus: States; r_ref output double; yawRateControl parameter double; car_params parameter double; r_lim output double; ay_max output double; settings parameter double
function [r_der_error,r_error, vx, r_ref,r_lim,ay_max]...
          = yawrate_reference(states, yawRateControl, car_params,settings)
      
%#codegen
r_lim = single(0);
ay_max = single(0);

delta = states.wheel_angle;
delta_der = states.wheel_speed;


% If Ku is negative there will be a problem if the denominator approaches
% zero at high speeds


%denominator = (car_params.l_f + car_params.l_r + car_params.Ku*states.V_x^2);
%r_ref = (states.V_x/(car_params.l_f + car_params.l_r + car_params.Ku*states.V_x^2))* delta;
L = single(1.5);
r_ref = (states.V_x/(L + yawRateControl.Ku*states.V_x^2))* delta;




%Fzi = [states.Fz_FL states.Fz_FR states.Fz_RL states.Fz_RR];
if yawRateControl.enable_r_ref_limit == 1
%     ay_max = (1/car_params.mass)*sqrt(max(0, sum(Fzi.*settings.mu_max_r)^2 - (car_params.mass*abs(states.ax))^2));
%     r_lim = (ay_max/abs(states.V_x))*sign(r_ref);
%     if abs(r_ref) > abs(r_lim) 
%         r_ref = r_lim;
%     end
    r_lim = settings.mu*yawRateControl.mu_scaling_r_ref_limit*9.81/states.V_x;
    if abs(r_ref) > abs(r_lim)
        r_ref = r_lim*sign(r_ref);
    end
end

r = states.r;
r_error = r_ref-r;

r_ref_der = (states.ax*delta + states.V_x*delta_der)/L;
r_der_error = r_ref_der*yawRateControl.ref_weight - states.r_der*yawRateControl.meas_weight;


vx = states.V_x;






%--------------------------%
%-----FEED FORWARD---------%
%--------------------------%

% Cornering Stiffnesses
% Cr = 26000;
% Cf = 26000;
% 
% lf = car_params.l_f;
% lr = car_params.l_r;
% Nbeta = lf*Cf - lr*Cr;
% Nr = (lf^2*Cf + lr^2*Cr)/states.V_x;
% Ndelta = -lf*Cf;
% Ybeta = Cf+Cr;
% Yr = (lf*Cf - lr*Cr)/states.V_x;
% Ydelta = -Cf;
% 
% C = car_params.mass*states.V_x*Nbeta + Nr*Ybeta - Nbeta*Yr;
% 
% E = Nbeta*Ydelta - Ndelta*Ybeta;
% F1 = -Ybeta;
% 
% Mz_FF = (C*r_ref/delta - E)*delta/(F1);

== matlab function CarMaker/Control_System /Control /Slip Rate Control /Traction Controllers/MATLAB Function1 ==
  data: states input Bus: States; SR_FL output double; SR_FR output double; SR_RL output double; SR_RR output double; T_req input double; tractionControl parameter double; Kp output double; Ki output double; settings parameter double; T_tv input Bus: Ti_lim
function [SR_FL,SR_FR,SR_RL,SR_RR, Kp, Ki] = slipRatioAndGains(states, T_req, tractionControl,settings,T_tv)
%#codegen


SR_FL = states.SR_FL;
SR_FR = states.SR_FR;
SR_RL = states.SR_RL;
SR_RR = states.SR_RR;

vx_kmh = states.V_x*3.6;

a_kp = single((tractionControl.Kp_end - tractionControl.Kp_start) / tractionControl.lookup_speed_end_kmh);
a_ki = single((tractionControl.Ki_end - tractionControl.Ki_start) / tractionControl.lookup_speed_end_kmh);


if ( ( (T_req + 0.0001) > 0) && (vx_kmh < tractionControl.full_gain_limit_kmh) )   
    Kp = min( (a_kp*max(0,vx_kmh) + tractionControl.Kp_start), tractionControl.Kp_end)  * abs(T_req)/(settings.max_motor_torque*4);
    Ki = min( (a_ki*max(0,vx_kmh) + tractionControl.Ki_start), tractionControl.Ki_end)  * abs(T_req)/(settings.max_motor_torque*4);
else
    Kp = min( (a_kp*max(0,vx_kmh) + tractionControl.Kp_start), tractionControl.Kp_end);
    Ki = min( (a_ki*max(0,vx_kmh) + tractionControl.Ki_start), tractionControl.Ki_end);
end






% This one solves starting from 0 kmh with the driver controlling the
% throttle. This statement reduces the gains according to the requested
% torque, to avoid oscillating torque output


% if ( ( (T_req + 0.0001) > 0) && (vx_kmh < tractionControl.full_gain_limit_kmh) )   
%     Kp_driving = min( (a_kp*max(0,vx_kmh) + tractionControl.Kp_start), tractionControl.Kp_end)  * abs(T_req)/(settings.max_motor_torque*4);
%     Ki_driving = min( (a_ki*max(0,vx_kmh) + tractionControl.Ki_start), tractionControl.Ki_end)  * abs(T_req)/(settings.max_motor_torque*4);
%     Kp_FL = Kp_driving;
%     Kp_FR = Kp_driving;
%     Kp_RL = Kp_driving;
%     Kp_RR = Kp_driving;
%     
%     Ki_FL = Ki_driving;
%     Ki_FR = Ki_driving;
%     Ki_RL = Ki_driving;
%     Ki_RR = Ki_driving;
%     %Kp = min( (a_kp*max(0,vx_kmh) + tractionControl.Kp_start), tractionControl.Kp_end)  * abs(T_req)/(settings.max_motor_torque*4);
%     %Ki = min( (a_ki*max(0,vx_kmh) + tractionControl.Ki_start), tractionControl.Ki_end)  * abs(T_req)/(settings.max_motor_torque*4);
% 
% % T_req positive and speed over full gain limit
% elseif ( ( (T_req + 0.0001) > 0) && (vx_kmh > tractionControl.full_gain_limit_kmh))
%     Kp_driving = min( (a_kp*max(0,vx_kmh) + tractionControl.Kp_start), tractionControl.Kp_end);
%     Ki_driving = min( (a_ki*max(0,vx_kmh) + tractionControl.Ki_start), tractionControl.Ki_end);
%     Kp_FL = Kp_driving;
%     Kp_FR = Kp_driving;
%     Kp_RL = Kp_driving;
%     Kp_RR = Kp_driving;
%     
%     Ki_FL = Ki_driving;
%     Ki_FR = Ki_driving;
%     Ki_RL = Ki_driving;
%     Ki_RR = Ki_driving;    
% else   
%     Kp_FL = min( (a_kp*max(0,vx_kmh) + tractionControl.Kp_start), tractionControl.Kp_end);
%     Kp_FR = min( (a_kp*max(0,vx_kmh) + tractionControl.Kp_start), tractionControl.Kp_end);
%     Kp_RL = min( (a_kp*max(0,vx_kmh) + tractionControl.Kp_start), tractionControl.Kp_end);
%     Kp_RR = min( (a_kp*max(0,vx_kmh) + tractionControl.Kp_start), tractionControl.Kp_end);
%     
%     Ki_FL = min( (a_ki*max(0,vx_kmh) + tractionControl.Ki_start), tractionControl.Ki_end);
%     Ki_FR = min( (a_ki*max(0,vx_kmh) + tractionControl.Ki_start), tractionControl.Ki_end);
%     Ki_RL = min( (a_ki*max(0,vx_kmh) + tractionControl.Ki_start), tractionControl.Ki_end);
%     Ki_RR = min( (a_ki*max(0,vx_kmh) + tractionControl.Ki_start), tractionControl.Ki_end);
%     
%     %Kp = tractionControl.Kp_braking;
%     %Ki = tractionControl.Ki_braking;
% end
% 
% if ( (T_tv.FL < 0) || (T_tv.FR < 0) || (T_tv.RL < 0) || (T_tv.RR < 0) )
%     Kp = tractionControl.Kp_braking;
%     Ki = tractionControl.Ki_braking;
% end

== matlab function CarMaker/Control_System /Output Interface /MATLAB Function ==
  data: Ti input Bus: Ti_lim; Ti_pos output Bus: Ti_pos; Ti_neg output Bus: Ti_neg; wi_setpoints output Bus: wi_set; settings parameter double; states input Bus: States; car_params parameter double
function [Ti_pos, Ti_neg, wi_setpoints] = setPointCalculation(Ti,settings,states,car_params)
%#codegen

% Conversion factor to calculate RPM limits based on speed limits
v_to_motor_RPM = single(60*car_params.GR/(2*pi*car_params.r_eff));

max_rpm = settings.max_RPM;
KERS_RPM_setpoint = settings.KERS_motor_RPM_setpoint;

% The RPM at which KERS is turned off
RPM_limit_low = settings.KERS_speed_limit_hyst_low*v_to_motor_RPM;

% The RPM at which KERS is allowed again
RPM_limit_high = settings.KERS_speed_limit_hyst_high*v_to_motor_RPM;


   persistent firstIteration;
   persistent KERS_ALLOWED_FL;
   persistent KERS_ALLOWED_FR;
   persistent KERS_ALLOWED_RL;
   persistent KERS_ALLOWED_RR;
   
   
   % Hysteresis on regenerative input based on RPM to avoid oscillation around 
   % allowed KERS RPM 
   if isempty(firstIteration)
      firstIteration = 2; % Avoid overflow in the register and count 1 again
      KERS_ALLOWED_FL = uint32(0);
      KERS_ALLOWED_FR = uint32(0);
      KERS_ALLOWED_RL = uint32(0);
      KERS_ALLOWED_RR = uint32(0);
   else
       
       %Hysteris around the minimum RPM Set point
       if     ( (KERS_ALLOWED_FL == 0) && (states.RPM_FL > RPM_limit_high) )
           KERS_ALLOWED_FL = uint32(1);
       elseif ( (KERS_ALLOWED_FL == 1) && (states.RPM_FL < RPM_limit_low) )
           KERS_ALLOWED_FL = uint32(0);
       end
       if     ( (KERS_ALLOWED_FR == 0) && (states.RPM_FR > RPM_limit_high) )
           KERS_ALLOWED_FR = uint32(1);
       elseif ( (KERS_ALLOWED_FR == 1) && (states.RPM_FR < RPM_limit_low) )
           KERS_ALLOWED_FR = uint32(0);
       end
       if     ( (KERS_ALLOWED_RL == 0) && (states.RPM_RL > RPM_limit_high) )
           KERS_ALLOWED_RL = uint32(1);
       elseif ( (KERS_ALLOWED_RL == 1) && (states.RPM_RL < RPM_limit_low) )
           KERS_ALLOWED_RL = uint32(0);
       end
       if     ( (KERS_ALLOWED_RR == 0) && (states.RPM_RR > RPM_limit_high) )
           KERS_ALLOWED_RR = uint32(1);
       elseif ( (KERS_ALLOWED_RR == 1) && (states.RPM_RR < RPM_limit_low) )
           KERS_ALLOWED_RR = uint32(0);
       end
       
       % Hysteresis around maximum RPM ? 
       
   end   
      
%***************** FL ************

if ( (Ti.FL <= 0) && (KERS_ALLOWED_FL == 1) ) 
    Ti_pos.FL = int16(0);
    Ti_neg.FL = int16( Ti.FL/car_params.Mn);
    wi_setpoints.FL = int16(KERS_RPM_setpoint);
elseif ( (Ti.FL <= 0) && (KERS_ALLOWED_FL == 0) )
    Ti_pos.FL = int16(0);
    Ti_neg.FL = int16(0);
    wi_setpoints.FL = int16(0);
elseif Ti.FL > 0
    Ti_pos.FL = int16( Ti.FL/car_params.Mn);
    Ti_neg.FL = int16(0);
    wi_setpoints.FL = int16(max_rpm);  
else
    Ti_pos.FL = int16(0);
    Ti_neg.FL = int16(0);
    wi_setpoints.FL = int16(0); 
end

%***************** FR ************

if ( (Ti.FR <= 0) && (KERS_ALLOWED_FR == 1) ) 
    Ti_pos.FR = int16(0);
    Ti_neg.FR = int16( Ti.FR/car_params.Mn);
    wi_setpoints.FR = int16(KERS_RPM_setpoint);
elseif ( (Ti.FR <= 0) && (KERS_ALLOWED_FR == 0) )
    Ti_pos.FR = int16(0);
    Ti_neg.FR = int16(0);
    wi_setpoints.FR = int16(0);
elseif Ti.FR > 0
    Ti_pos.FR = int16( Ti.FR/car_params.Mn);
    Ti_neg.FR = int16(0);
    wi_setpoints.FR = int16(max_rpm);  
else
    Ti_pos.FR = int16(0);
    Ti_neg.FR = int16(0);
    wi_setpoints.FR = int16(0); 
end
%***************** RL ************
if ( (Ti.RL <= 0) && (KERS_ALLOWED_RL == 1) ) 
    Ti_pos.RL = int16(0);
    Ti_neg.RL = int16( Ti.RL/car_params.Mn);
    wi_setpoints.RL = int16(KERS_RPM_setpoint);
elseif ( (Ti.RL <= 0) && (KERS_ALLOWED_RL == 0) )
    Ti_pos.RL = int16(0);
    Ti_neg.RL = int16(0);
    wi_setpoints.RL = int16(0);
elseif Ti.RL > 0
    Ti_pos.RL = int16( Ti.RL/car_params.Mn);
    Ti_neg.RL = int16(0);
    wi_setpoints.RL = int16(max_rpm);  
else
    Ti_pos.RL = int16(0);
    Ti_neg.RL = int16(0);
    wi_setpoints.RL = int16(0); 
end

%***************** RR ************
if ( (Ti.RR <= 0) && (KERS_ALLOWED_RR == 1) ) 
    Ti_pos.RR = int16(0);
    Ti_neg.RR = int16( Ti.RR/car_params.Mn);
    wi_setpoints.RR = int16(KERS_RPM_setpoint);
elseif ( (Ti.RR <= 0) && (KERS_ALLOWED_RR == 0) )
    Ti_pos.RR = int16(0);
    Ti_neg.RR = int16(0);
    wi_setpoints.RR = int16(0);
elseif Ti.RR > 0
    Ti_pos.RR = int16( Ti.RR/car_params.Mn);
    Ti_neg.RR = int16(0);
    wi_setpoints.RR = int16(max_rpm);  
else
    Ti_pos.RR = int16(0);
    Ti_neg.RR = int16(0);
    wi_setpoints.RR = int16(0); 
end

end

== matlab function CarMaker/Control_System /OutputTelemetri ==
  data: states input double; OutputTelemetri_control output Bus: OutputTelemetri_Control; T_req input double; r_ref input double; Mz_ref input double
function OutputTelemetri_control = OutputTelemetri(states, T_req, r_ref, Mz_ref)
%#codegen

OutputTelemetri_control.T_req   = T_req;
OutputTelemetri_control.Mz_ref  = Mz_ref;
OutputTelemetri_control.r_ref   = r_ref;

== matlab function CarMaker/Estimations/Fz_Estimation/FzEstLoadTransfer ==
  data: Fz_loadTransfer_est output Bus: normalForces; sensor input Bus: SensorInputs; car_params parameter double; vx input double
function Fz_loadTransfer_est  = FzEstLoadTransfer(sensor,car_params,vx)
%#codegen




mv = car_params.car_mass + car_params.driver_mass; % Total mass( driver + car) X
l  = car_params.l; %Wheel base X
lr = car_params.l_r; % X
lf = car_params.l_f;% X

ef = car_params.t_f*2; % Front track X
er = car_params.t_r*2; % Rear track X


hc = car_params.CoG_height; % X
g = 9.81; % X
air_density = single(1.2);

Fz_loadTransfer_est.FL = (0.5*mv*(lr*g/l - hc*sensor.ax/l) - mv*(lr*g/l - hc*sensor.ax/l)*hc*sensor.ay/(ef*g))  + (vx^2 * car_params.aero_ref_area* car_params.aero_lift_coeff*air_density)/8;
Fz_loadTransfer_est.FR = (0.5*mv*(lr*g/l - hc*sensor.ax/l) + mv*(lr*g/l - hc*sensor.ax/l)*hc*sensor.ay/(ef*g))  + (vx^2 * car_params.aero_ref_area* car_params.aero_lift_coeff*air_density)/8;
Fz_loadTransfer_est.RL = (0.5*mv*(lf*g/l + hc*sensor.ax/l) - mv*(lf*g/l + hc*sensor.ax/l)*hc*sensor.ay/(er*g))  + (vx^2 * car_params.aero_ref_area* car_params.aero_lift_coeff*air_density)/8;
Fz_loadTransfer_est.RR = (0.5*mv*(lf*g/l + hc*sensor.ax/l) + mv*(lf*g/l + hc*sensor.ax/l)*hc*sensor.ay/(er*g))  + (vx^2 * car_params.aero_ref_area* car_params.aero_lift_coeff*air_density)/8;

end

== matlab function CarMaker/Sensors /"Measured Power"/MATLAB Function ==
  data: RPM_FL_IN input double; RPM_FR_IN input double; RPM_RL_IN input double; RPM_RR_IN input double; Pm_FL output double; T input double; T_FL output double; RPM_FL output double; Pm_FR output double; T_FR output double; RPM_FR output double; Pm_RL output double; T_RL output double; RPM_RL output double; Pm_RR output double; T_RR output double; RPM_RR output double
function [Pm_FL, T_FL, RPM_FL,Pm_FR, T_FR, RPM_FR,Pm_RL, T_RL,...
          RPM_RL,Pm_RR, T_RR, RPM_RR] = powerMeasurement(RPM_FL_IN, RPM_FR_IN,RPM_RL_IN,RPM_RR_IN, T)
%#codegen

%Conversion from RPM to rad/s
c = single(2*pi/60);

T_FL = T.FL;
T_FR = T.FR;
T_RL = T.RL;
T_RR = T.RR;
RPM_FL = RPM_FL_IN;
RPM_FR = RPM_FR_IN;
RPM_RL = RPM_RL_IN;
RPM_RR = RPM_RR_IN;


Pm_FL = RPM_FL*c*T.FL;
Pm_FR = RPM_FR*c*T.FR;
Pm_RL = RPM_RL*c*T.RL;
Pm_RR = RPM_RR*c*T.RR;

== matlab function CarMaker/Control_System /Control /Torque allocation /MATLAB Function ==
  data: states input double; maxMotorTorque output Bus: maxMotorTorque; settings parameter double
function maxMotorTorque = findMaxMotorTorque(states,settings)
%#codegen

% DC Voltage
% Max allowable current draw in total
% Load distribution

Fzi = [max(1,states.Fz_FL) max(1,states.Fz_FR) max(1,states.Fz_RL) max(1,states.Fz_RR)]';

switch settings.TV_Method
    case 1 % No negative torque
        alfa_r =  (Fzi(3) + Fzi(4)) / (Fzi(1) + Fzi(2) + Fzi(3) + Fzi(4));
    case 2 % with negative torque
        alfa_r =  (Fzi(3) + Fzi(4)) / (Fzi(1) + Fzi(2) + Fzi(3) + Fzi(4));
    case 3 % static 25 %
        alfa_r = single(0.5);
    case 4 % with negative torque, no Fz
        alfa_r = single(0.5);
    otherwise
        alfa_r = single(0.5);
end

        
        


DC_voltage = states.DC_voltage;
max_discharge = settings.max_battery_discharge;


max_torque_front = min(min(settings.max_motor_torque,(DC_voltage*max_discharge*(1-alfa_r))/(2*max(1,states.RPM_FL)*2*pi/60)) , ...
                           (min(settings.max_motor_torque,(DC_voltage*max_discharge*(1-alfa_r))/(2*max(1,states.RPM_FR)*2*pi/60))));
                       
max_torque_rear = min(min(settings.max_motor_torque,(DC_voltage*max_discharge*(1-alfa_r))/(2*max(1,states.RPM_RL)*2*pi/60)) , ...
                           (min(settings.max_motor_torque,(DC_voltage*max_discharge*(1-alfa_r))/(2*max(1,states.RPM_RR)*2*pi/60))));                     
                       
maxMotorTorque.mmt_FL = max_torque_front;
maxMotorTorque.mmt_FR = max_torque_front;
maxMotorTorque.mmt_RL = max_torque_rear;
maxMotorTorque.mmt_RR = max_torque_rear;

                       
%maxMotorTorque.mmt_FR = min(settings.max_motor_torque,(DC_voltage*max_discharge*(1-alfa_r))/(2*max(1,states.RPM_FR)*2*pi/60));
%maxMotorTorque.mmt_RL = min(settings.max_motor_torque,(DC_voltage*max_discharge*(alfa_r))/(2*max(1,states.RPM_RL)*2*pi/60));
%maxMotorTorque.mmt_RR = min(settings.max_motor_torque,(DC_voltage*max_discharge*(alfa_r))/(2*max(1,states.RPM_RR)*2*pi/60));
